simulink model "simulation_part2"  (R2014b)
settings: Solver=ode45  StartTime=0.0  StopTime=20  RelTol=1e-3
values from neighbouring files (symbols this model uses):
  c1 = 0.01    [Variables_part2.m]
  c2 = 0.01    [Variables_part2.m]
  g = 9.81    [Variables_part2.m]
  J = M*L^2+m*l^2    (= 76.8)    [Variables_part2.m]
  k_bemf = 0.5    [Variables_part2.m]
  k_t = 0.75    [Variables_part2.m]
  L = 0.4    [Variables_part2.m]
  l = 1    [Variables_part2.m]
  M = 55    [Variables_part2.m]
  m = 68    [Variables_part2.m]
  R = 0.5    [Variables_part2.m]
  r_a = 1.4    [Variables_part2.m]
libraries: simulink x2
settings Model: Creator=hchiang  LastModifiedBy=hchiang

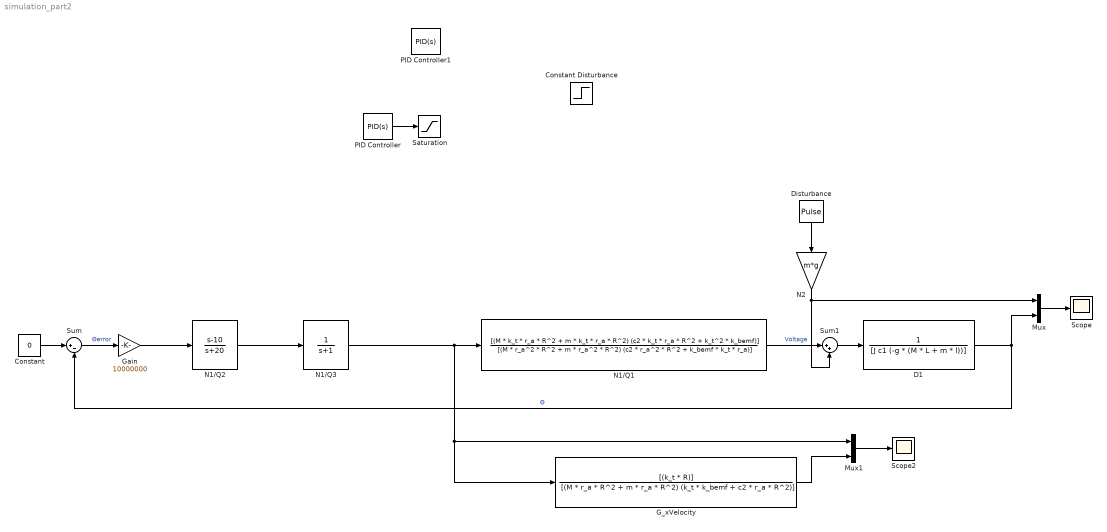
== system simulation_part2 ==
  Constant : Constant  Value=0
  Constant Disturbance : Step  SampleTime=0
  D1 : TransferFcn  Denominator=[J c1 (-g * (M * L + m * l))]
  Disturbance : DiscretePulseGenerator  PulseType=Time based  Amplitude=.01  Period=100  PhaseDelay=1
  G_xVelocity : TransferFcn  Numerator=[(k_t * R)]  Denominator=[(M * r_a * R^2 + m * r_a * R^2) (k_t * k_bemf + c2 * r_a * R^2)]
  Gain : Gain  Gain=10000000
  Mux : Mux  Inputs=2
  Mux1 : Mux  Inputs=2
  N1/Q1 : TransferFcn  Numerator=[(M * k_t * r_a * R^2 + m * k_t * r_a * R^2) (c2 * k_t * r_a * R^2 + k_t^2 * k_bemf)]  Denominator=[(M * r_a^2 * R^2 + m * r_a^2 * R^2) (c2 * r_a^2 * R^2 + k_bemf * k_t * r_a)]
  N1/Q2 : TransferFcn  Numerator=[1 -10]  Denominator=[1 20]
  N1/Q3 : TransferFcn  Denominator=[1 1]
  N2 : Gain  Gain=m*g
  PID Controller : simulink/Continuous/PID Controller  Controller=PID  TimeDomain=Continuous-time  SampleTime=-1  IntegratorMethod=Forward Euler  FilterMethod=Forward Euler  Form=Parallel  P=1750  I=14  D=189  N=100  InitialConditionSource=internal  InitialConditionForIntegrator=0  InitialConditionForFilter=0  ExternalReset=none  LimitOutput=off  UpperSaturationLimit=inf  LowerSaturationLimit=-inf  LinearizeAsGain=on  AntiWindupMode=none  Kb=1  TrackingMode=off  Kt=1  PParamMin=[]  PParamMax=[]  IParamMin=[]  IParamMax=[]  DParamMin=[]  DParamMax=[]  NParamMin=[]  NParamMax=[]  KbParamMin=[]  KbParamMax=[]  KtParamMin=[]  KtParamMax=[]  POutMin=[]  POutMax=[]  IOutMin=[]  IOutMax=[]  DOutMin=[]  DOutMax=[]  NOutMin=[]  NOutMax=[]  KbOutMin=[]  KbOutMax=[]  KtOutMin=[]  KtOutMax=[]  IntegratorOutMin=[]  IntegratorOutMax=[]  FilterOutMin=[]  FilterOutMax=[]  SumOutMin=[]  SumOutMax=[]  SumI1OutMin=[]  SumI1OutMax=[]  SumI2OutMin=[]  SumI2OutMax=[]  SumI3OutMin=[]  SumI3OutMax=[]  SumDOutMin=[]  SumDOutMax=[]  SaturationOutMin=[]  SaturationOutMax=[]  IntegratorContinuousStateAttributes=''  IntegratorStateMustResolveToSignalObject=off  IntegratorRTWStateStorageClass=Auto  FilterContinuousStateAttributes=''  FilterStateMustResolveToSignalObject=off  FilterRTWStateStorageClass=Auto  DifferentiatorICPrevScaledInput=0  DifferentiatorOutMin=[]  DifferentiatorOutMax=[]  UseFilter=on
  PID Controller1 : simulink/Continuous/PID Controller  Controller=PID  TimeDomain=Continuous-time  SampleTime=-1  IntegratorMethod=Forward Euler  FilterMethod=Forward Euler  Form=Parallel  P=1800  I=20  D=80  N=100  InitialConditionSource=internal  InitialConditionForIntegrator=0  InitialConditionForFilter=0  ExternalReset=none  LimitOutput=off  UpperSaturationLimit=inf  LowerSaturationLimit=-inf  LinearizeAsGain=on  AntiWindupMode=none  Kb=1  TrackingMode=off  Kt=1  PParamMin=[]  PParamMax=[]  IParamMin=[]  IParamMax=[]  DParamMin=[]  DParamMax=[]  NParamMin=[]  NParamMax=[]  KbParamMin=[]  KbParamMax=[]  KtParamMin=[]  KtParamMax=[]  POutMin=[]  POutMax=[]  IOutMin=[]  IOutMax=[]  DOutMin=[]  DOutMax=[]  NOutMin=[]  NOutMax=[]  KbOutMin=[]  KbOutMax=[]  KtOutMin=[]  KtOutMax=[]  IntegratorOutMin=[]  IntegratorOutMax=[]  FilterOutMin=[]  FilterOutMax=[]  SumOutMin=[]  SumOutMax=[]  SumI1OutMin=[]  SumI1OutMax=[]  SumI2OutMin=[]  SumI2OutMax=[]  SumI3OutMin=[]  SumI3OutMax=[]  SumDOutMin=[]  SumDOutMax=[]  SaturationOutMin=[]  SaturationOutMax=[]  IntegratorContinuousStateAttributes=''  IntegratorStateMustResolveToSignalObject=off  IntegratorRTWStateStorageClass=Auto  FilterContinuousStateAttributes=''  FilterStateMustResolveToSignalObject=off  FilterRTWStateStorageClass=Auto  DifferentiatorICPrevScaledInput=0  DifferentiatorOutMin=[]  DifferentiatorOutMax=[]  UseFilter=on
  Saturation : Saturate  UpperLimit=10  LowerLimit=-10
  Scope : Scope
      settings: TimeRange=80.4733727810651  YMin=-1.506578947368418  YMax=0.7960526315789487
  Scope2 : Scope
      settings: TimeRange=10  YMin=-1  YMax=1  SaveName=ScopeData2
  Sum : Sum  Inputs=|+-
  Sum1 : Sum  Inputs=|++
  wires:
  N1/Q1/1 -> Sum1/1  "Voltage"
  N2/1 -> Sum1/2, Mux/1
  Constant/1 -> Sum/1
  Sum1/1 -> D1/1
  D1/1 -> Sum/2, Mux/2  "Θ"
  Mux/1 -> Scope/1
  Sum/1 -> Gain/1  "Θerror"
  Mux1/1 -> Scope2/1
  G_xVelocity/1 -> Mux1/2
  Disturbance/1 -> N2/1
  PID Controller/1 -> Saturation/1
  Gain/1 -> N1/Q2/1
  N1/Q2/1 -> N1/Q3/1
  N1/Q3/1 -> N1/Q1/1, G_xVelocity/1, Mux1/1
